simulink model "RI_EGH_ISZM_DI"  (R2013b)
settings: Solver=ode45  StartTime=0.0  StopTime=75e-3  MaxStep=tau_RL/10/25  RelTol=1e-3
InitFcn:
  | % Villamos áramköri rész
  | R = 1.76;
  | L = 658e-6;
  | 
  | % Mágneskör
  | k_T = 68.3e-3;
  | k_E = 68.3e-3;
  | 
  | % Forgó részrendszer
  | J = 99.5e-7;
  | B = 5.7301e-6;
  | 
  | % A belső áramszabályzókör hangolása
  | K_RL = 1/R;
  | tau_RL = L/R;
  | 
  | % ZPK
  | T_I_RL_ZPK = tau_RL;
  | K_PI_RL_ZPK = 1/K_RL * 10;
  | 
  | % MRZK
  | xi_CL_RL = 1;
  | tau_CL_RL = tau_RL/10;
  | 
  | K_PI_RL_MRZK = (2*xi_CL_RL*tau_RL - tau_CL_RL)/(K_RL*tau_CL_RL);
  | T_I_RL_MRZK = (2*xi_CL_RL*tau_RL - tau_CL_RL)*tau_CL_RL/tau_RL;
  | 
  | % A külső szögsebesség-szabályzókör hangolása
  | K_JB = k_T/B;
  | tau_JB = J/B;
  | 
  | % ZPK
  | T_I_JB_ZPK = tau_JB;
  | K_PI_JB_ZPK = 1/K_JB * 2000;
  | 
  | % MRZK
  | xi_CL_JB = 2;
  | tau_CL_JB = tau_JB/2000;
  | 
  | K_PI_JB_MRZK = (2*xi_CL_JB*tau_JB - tau_CL_JB)/(K_JB*tau_CL_JB);
  | T_I_JB_MRZK = (2*xi_CL_JB*tau_JB - tau_CL_JB)*tau_CL_JB/tau_JB;
libraries: RI_MK x4
settings Model: Creator=Szalay  LastModifiedBy=Szalay

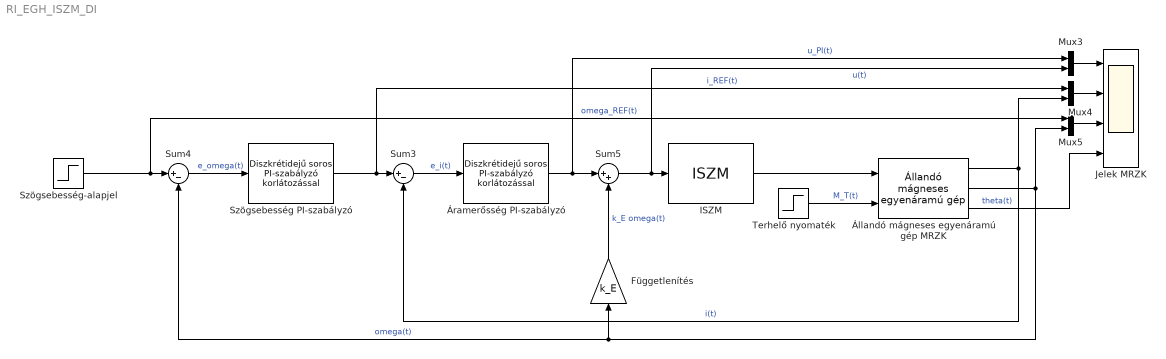
== system RI_EGH_ISZM_DI ==
  Függetlenítés : Gain  Gain=k_E
  ISZM : RI_MK/ISZM  U_T=48  f_ISZM=25000  T_S=400e-9
  Jelek MRZK : Scope  NumInputPorts=4
      settings: ShowLegends=on  TimeRange=0.08  YMin=-50~-5~-50~-0.1  YMax=50~5~300~0.7000000000000001
  Mux3 : Mux  Inputs=2
  Mux4 : Mux  Inputs=2
  Mux5 : Mux  Inputs=2
  Sum3 : Sum  Inputs=|+-
  Sum4 : Sum  Inputs=|+-
  Sum5 : Sum  Inputs=|++
  Szögsebesség PI-szabályzó : RI_MK/Diszkrétidejű soros PI-szabályzó korlátozással  K_PI=1  T_I=1  L_U=5  L_L=-5  T_T=1  T_S=1/25000
  Szögsebesség-alapjel : Step  Time=10e-3  After=300  SampleTime=0
  Terhelő nyomaték : Step  Time=50e-3  After=100e-3  SampleTime=0
  Állandó mágneses egyenáramú gép MRZK : RI_MK/Állandó mágneses egyenáramú gép  R=R  L=L  k_T=k_T  k_E=k_E  J=J  B=B  i_0=0  omega_0=0  theta_0=0
  Áramerősség PI-szabályzó : RI_MK/Diszkrétidejű soros PI-szabályzó korlátozással  K_PI=K_PI_RL_MRZK  T_I=T_I_RL_MRZK  L_U=48  L_L=-48  T_T=T_I_RL_MRZK  T_S=1/25000
  wires:
  Sum4/1 -> Szögsebesség PI-szabályzó/1  "e_omega(t)"
  Szögsebesség PI-szabályzó/1 -> Mux4/1, Sum3/1  "i_REF(t)"
  Sum3/1 -> Áramerősség PI-szabályzó/1  "e_i(t)"
  Áramerősség PI-szabályzó/1 -> Mux3/1, Sum5/1  "u_PI(t)"
  Sum5/1 -> ISZM/1, Mux3/2  "u(t)"
  Állandó mágneses egyenáramú gép MRZK/1 -> Mux4/2, Sum3/2  "i(t)"
  Állandó mágneses egyenáramú gép MRZK/2 -> Mux5/2, Sum4/2, Függetlenítés/1  "omega(t)"
  Függetlenítés/1 -> Sum5/2  "k_E omega(t)"
  Szögsebesség-alapjel/1 -> Mux5/1, Sum4/1  "omega_REF(t)"
  Mux3/1 -> Jelek MRZK/1
  Mux4/1 -> Jelek MRZK/2
  Mux5/1 -> Jelek MRZK/3
  Állandó mágneses egyenáramú gép MRZK/3 -> Jelek MRZK/4  "theta(t)"
  Terhelő nyomaték/1 -> Állandó mágneses egyenáramú gép MRZK/2  "M_T(t)"
  ISZM/1 -> Állandó mágneses egyenáramú gép MRZK/1
